simulink model "yangji"  (R2023a)
settings: Solver=VariableStepAuto  StartTime=0.0  StopTime=10.0  RelTol=1e-3
settings Model: Creator=Administrator  LastModifiedBy=Administrator

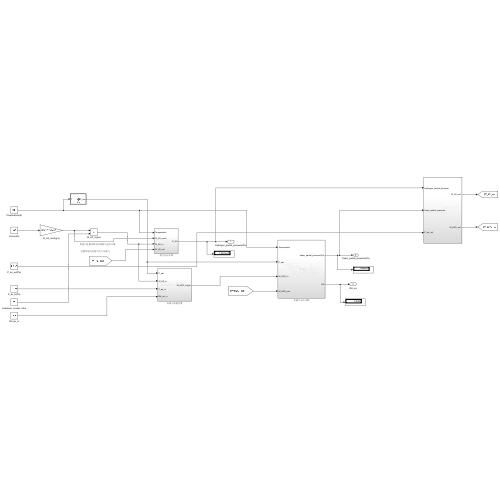
[thumbnail: Simulink's stored preview of the top-level diagram]
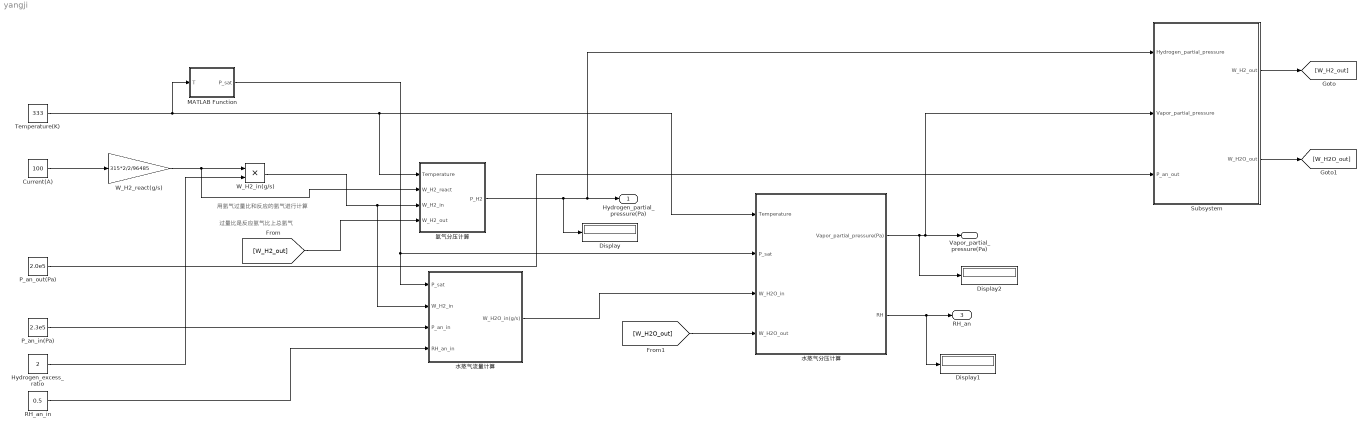
== system yangji ==
  note: 过量比是反应氢气比上总氢气
  note: 用氢气过量比和反应的氢气进行计算
  Current(A) : Constant  Value=100
  Display : Display
  Display1 : Display
  Display2 : Display
  Hydrogen_excess_ratio : Constant  Value=2
  MATLAB Function : MATLAB Function  TreatAsAtomicUnit=on
  P_an_in(Pa) : Constant  Value=2.3e5
  P_an_out(Pa) : Constant  Value=2.0e5
  RH_an_in : Constant  Value=0.5
  Subsystem : Subsystem
  Temperature(K) : Constant  Value=333
  W_H2_in(g/s) : Product
  W_H2_react(g/s) : Gain  Gain=315*2/2/96485
  氢气分压计算 : Subsystem
  水蒸气分压计算 : Subsystem
  水蒸气流量计算 : Subsystem
  Hydrogen_partial_pressure(Pa) : Outport
  Vapor_partial_pressure(Pa) : Outport  Port=2
  RH_an : Outport  Port=3
  wires:
  Current(A)/1 -> W_H2_react(g/s)/1
  W_H2_react(g/s)/1 -> 氢气分压计算/2(W_H2_react), W_H2_in(g/s)/1
  Hydrogen_excess_ratio/1 -> W_H2_in(g/s)/2
  Temperature(K)/1 -> MATLAB Function/1(T), 水蒸气分压计算/1(Temperature), 氢气分压计算/1(Temperature)
  W_H2_in(g/s)/1 -> 水蒸气流量计算/2(W_H2_in), 氢气分压计算/3(W_H2_in)
  [W_H2_out] -> 氢气分压计算/4(W_H2_out)
  氢气分压计算/1(P_H2) -> Display/1, Subsystem/1(Hydrogen_partial_pressure), Hydrogen_partial_pressure(Pa)/1
  MATLAB Function/1(P_sat) -> 水蒸气流量计算/1(P_sat), 水蒸气分压计算/2(P_sat)
  P_an_in(Pa)/1 -> 水蒸气流量计算/3(P_an_in)
  RH_an_in/1 -> 水蒸气流量计算/4(RH_an_in)
  水蒸气流量计算/1(W_H2O_in(g/s)) -> 水蒸气分压计算/3(W_H2O_in)
  [W_H2O_out] -> 水蒸气分压计算/4(W_H2O_out)
  水蒸气分压计算/1(Vapor_partial_pressure(Pa)) -> Display2/1, Subsystem/2(Vapor_partial_pressure), Vapor_partial_pressure(Pa)/1
  水蒸气分压计算/2(RH) -> Display1/1, RH_an/1
  P_an_out(Pa)/1 -> Subsystem/3(P_an_out)
  Subsystem/1("W_H2_out ") -> [W_H2_out]
  Subsystem/2("W_H2O_out ") -> [W_H2O_out]

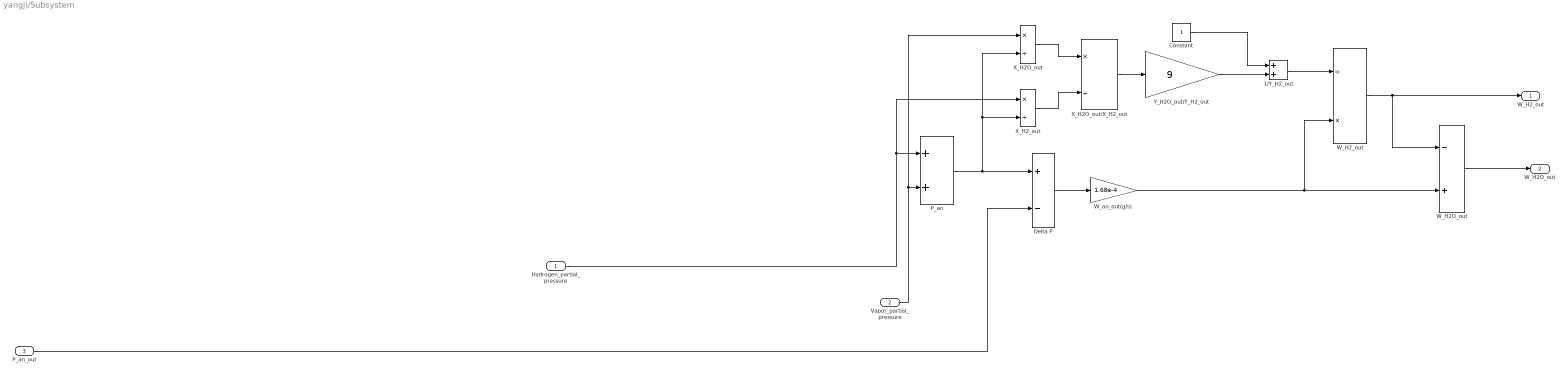
== system yangji/Subsystem ==
  Hydrogen_partial_pressure : Inport
  Vapor_partial_pressure : Inport  Port=2
  P_an_out : Inport  Port=3
  1/Y_H2_out : Sum
  Constant : Constant
  Delta P : Sum  Inputs=+-
  P_an : Sum
  W_H2O_out : Sum  Inputs=-+
  W_H2_out : Product  Inputs=/*
  W_an_out(g/s) : Gain  Gain=1.68e-4
  X_H2O_out : Product  Inputs=*/
  X_H2O_out/X_H2_out : Product  Inputs=*/
  X_H2_out : Product  Inputs=*/
  Y_H2O_out/Y_H2_out : Gain  Gain=9
  "W_H2_out " : Outport
  "W_H2O_out " : Outport  Port=2
  wires:
  X_H2_out/1 -> X_H2O_out/X_H2_out/2
  Y_H2O_out/Y_H2_out/1 -> 1/Y_H2_out/2
  P_an/1 -> X_H2O_out/2, X_H2_out/2, Delta P/1
  X_H2O_out/X_H2_out/1 -> Y_H2O_out/Y_H2_out/1
  Hydrogen_partial_pressure/1 -> X_H2_out/1, P_an/1
  W_H2_out/1 -> "W_H2_out "/1, W_H2O_out/1
  W_an_out(g/s)/1 -> W_H2_out/2, W_H2O_out/2
  Delta P/1 -> W_an_out(g/s)/1
  Constant/1 -> 1/Y_H2_out/1
  P_an_out/1 -> Delta P/2
  X_H2O_out/1 -> X_H2O_out/X_H2_out/1
  Vapor_partial_pressure/1 -> X_H2O_out/1, P_an/2
  1/Y_H2_out/1 -> W_H2_out/1
  W_H2O_out/1 -> "W_H2O_out "/1

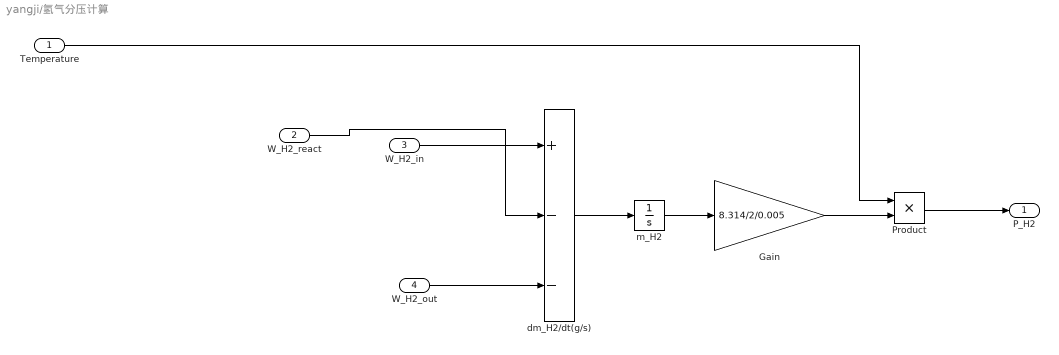
== system yangji/氢气分压计算 ==
  Temperature : Inport
  W_H2_react : Inport  Port=2
  W_H2_in : Inport  Port=3
  W_H2_out : Inport  Port=4
  Gain : Gain  Gain=8.314/2/0.005
  Product : Product
  dm_H2/dt(g/s) : Sum  Inputs=+--
  m_H2 : Integrator  InitialCondition=0.01
  P_H2 : Outport
  wires:
  Temperature/1 -> Product/1
  m_H2/1 -> Gain/1
  Gain/1 -> Product/2
  W_H2_in/1 -> dm_H2/dt(g/s)/1
  W_H2_out/1 -> dm_H2/dt(g/s)/3
  dm_H2/dt(g/s)/1 -> m_H2/1
  Product/1 -> P_H2/1
  W_H2_react/1 -> dm_H2/dt(g/s)/2

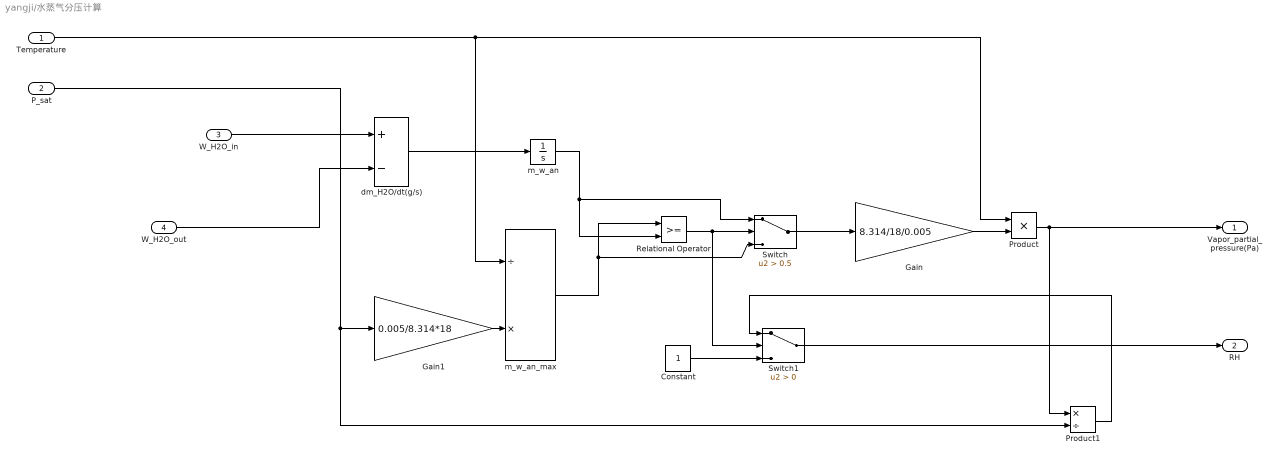
== system yangji/水蒸气分压计算 ==
  Temperature : Inport
  P_sat : Inport  Port=2
  W_H2O_in : Inport  Port=3
  W_H2O_out : Inport  Port=4
  Constant : Constant
  Gain : Gain  Gain=8.314/18/0.005
  Gain1 : Gain  Gain=0.005/8.314*18
  Product : Product
  Product1 : Product  Inputs=*/
  Relational Operator : RelationalOperator  OutDataTypeStr=boolean  RndMeth=Simplest  InputSameDT=off
  Switch : Switch  Criteria=u2 > Threshold  Threshold=0.5  SaturateOnIntegerOverflow=off  InputSameDT=off
  Switch1 : Switch  Criteria=u2 > Threshold  SaturateOnIntegerOverflow=off  InputSameDT=off
  dm_H2O/dt(g/s) : Sum  Inputs=+-
  m_w_an : Integrator  InitialCondition=0.01
  m_w_an_max : Product  Inputs=/*
  Vapor_partial_pressure(Pa) : Outport
  RH : Outport  Port=2
  wires:
  m_w_an_max/1 -> Relational Operator/1, Switch/3
  Temperature/1 -> Product/1, m_w_an_max/1
  m_w_an/1 -> Switch/1, Relational Operator/2
  Switch/1 -> Gain/1
  dm_H2O/dt(g/s)/1 -> m_w_an/1
  Product/1 -> Vapor_partial_pressure(Pa)/1, Product1/1
  Gain1/1 -> m_w_an_max/2
  Constant/1 -> Switch1/3
  Relational Operator/1 -> Switch1/2, Switch/2
  Gain/1 -> Product/2
  Product1/1 -> Switch1/1
  W_H2O_in/1 -> dm_H2O/dt(g/s)/1
  Switch1/1 -> RH/1
  P_sat/1 -> Product1/2, Gain1/1
  W_H2O_out/1 -> dm_H2O/dt(g/s)/2

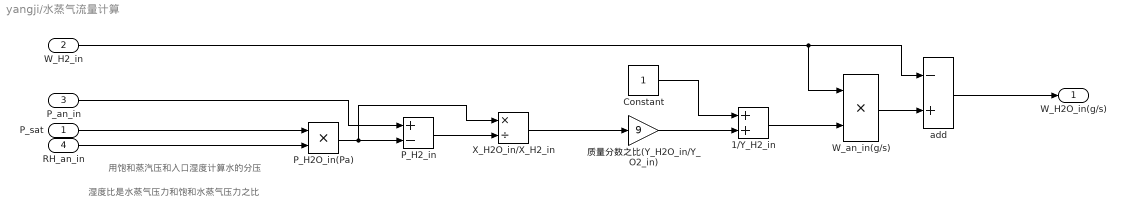
== system yangji/水蒸气流量计算 ==
  note: 湿度比是水蒸气压力和饱和水蒸气压力之比
  note: 用饱和蒸汽压和入口湿度计算水的分压
  P_sat : Inport
  W_H2_in : Inport  Port=2
  P_an_in : Inport  Port=3
  RH_an_in : Inport  Port=4
  1/Y_H2_in : Sum
  Constant : Constant
  P_H2O_in(Pa) : Product
  P_H2_in : Sum  Inputs=+-
  W_an_in(g/s) : Product
  X_H2O_in/X_H2_in : Product  Inputs=*/
  add : Sum  Inputs=-+
  质量分数之比(Y_H2O_in/Y_O2_in) : Gain  Gain=9
  W_H2O_in(g/s) : Outport
  wires:
  W_an_in(g/s)/1 -> add/2
  1/Y_H2_in/1 -> W_an_in(g/s)/2
  质量分数之比(Y_H2O_in/Y_O2_in)/1 -> 1/Y_H2_in/2
  W_H2_in/1 -> W_an_in(g/s)/1, add/1
  P_sat/1 -> P_H2O_in(Pa)/1
  X_H2O_in/X_H2_in/1 -> 质量分数之比(Y_H2O_in/Y_O2_in)/1
  P_H2O_in(Pa)/1 -> X_H2O_in/X_H2_in/1, P_H2_in/2
  Constant/1 -> 1/Y_H2_in/1
  P_H2_in/1 -> X_H2O_in/X_H2_in/2
  add/1 -> W_H2O_in(g/s)/1
  RH_an_in/1 -> P_H2O_in(Pa)/2
  P_an_in/1 -> P_H2_in/1

== matlab function yangji/MATLAB Function ==
  data: T input; P_sat output
function P_sat = fcn(T)

P_sat = exp(23.196-3816.44/(T-46.13));
